simulink model "imcpendel3"  (R2021b)
settings: Solver=ode15s  StartTime=0.0  StopTime=1000  RelTol=1e-3
values from neighbouring files (symbols this model uses):
  A = double(A)    [Eindampfanlage.m]
  B = double(B)    [Eindampfanlage.m]
  C = double(C)    [Eindampfanlage.m]
  D = zeros(p,m)    [Eindampfanlage.m]
  xR = [1; 15; 70]    [Eindampfanlage.m]
settings Model: Creator=mluser  LastModifiedBy=1star
settings DebuggingCC: UnconnectedInputMsg=none  UnconnectedOutputMsg=none  UnconnectedLineMsg=none
settings ModelReferenceCC: EnableRefExpFcnMdlSchedulingChecks=off
settings RTWCC: DLArmComputeVersion=20.02.1

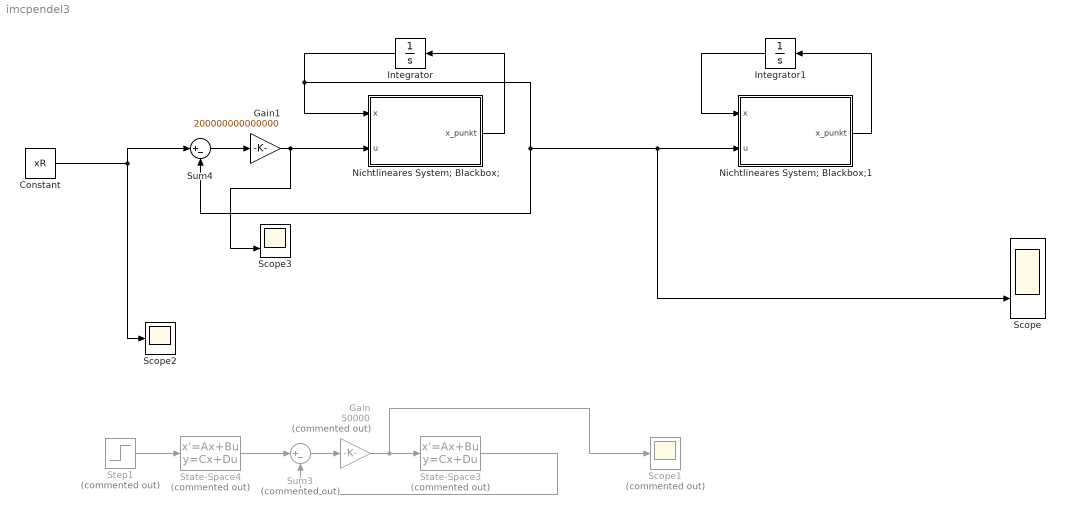
== system imcpendel3 ==
  Constant : Constant  Value=xR
  Gain : Gain  Commented=on  Gain=50000
  Gain1 : Gain  Gain=200000000000000
  Integrator : Integrator  InitialCondition=xR
  Integrator1 : Integrator  InitialCondition=xR
  Nichtlineares System; Blackbox; : MATLAB Function
  Nichtlineares System; Blackbox;1 : MATLAB Function
  Scope : Scope  NumInputPorts=2
  Scope1 : Scope  Commented=on
  Scope2 : Scope
  Scope3 : Scope  NumInputPorts=2
  State-Space3 : StateSpace  Commented=on  A=A  B=B  C=C  D=D  InitialCondition=0
  State-Space4 : StateSpace  Commented=on  A=A  B=B  C=C  D=D  InitialCondition=0
  Step1 : Step  Commented=on  SampleTime=0
  Sum3 : Sum  Commented=on  Inputs=|+-
  Sum4 : Sum  Inputs=|+-
  wires:
  State-Space3/1 -> Sum3/2
  Step1/1 -> State-Space4/1
  State-Space4/1 -> Sum3/1
  Gain/1 -> Scope1/1, State-Space3/1
  Sum3/1 -> Gain/1
  Nichtlineares System; Blackbox;/1(x_punkt) -> Integrator/1
  Constant/1 -> Scope2/1, Sum4/1
  Sum4/1 -> Gain1/1
  Gain1/1 -> Scope3/2, Nichtlineares System; Blackbox;/2(u)
  Integrator/1 -> Scope/2, Nichtlineares System; Blackbox;1/2(u), Sum4/2, Nichtlineares System; Blackbox;/1(x)
  Nichtlineares System; Blackbox;1/1(x_punkt) -> Integrator1/1
  Integrator1/1 -> Nichtlineares System; Blackbox;1/1(x)

== matlab function imcpendel3/Nichtlineares System; Blackbox; ==
  data: x input; x_punkt output; u input
function x_punkt = fcn(x, u)
a1 = 0.00751;
a2 = 0.00418;
a3 = 0.05;
a4 = 0.03755;
a5 = 0.02091;
a6 = 0.00315;

b1 = 0.00192;
b2 = 0.05;
b3 = 0.00959;
b4 = 0.1866;
b5 = 0.14;

k1 = 0.01061;
k2 = 2.5;
k3 = 6.84;
k4 = 2.5531;

x1_punkt = a1*x(3)+a2*x(2)-b1*u(1)-b2*u(2)-k1;
x2_punkt = -a3*x(2)*u(2)+k2;
x3_punkt = -a4*x(3)-a5*x(2)+b3*u(1)-(a6*x(3)+b4)*u(3)/(b5*u(3)+k3)+k4;

x_punkt = [x1_punkt;x2_punkt;x3_punkt];

== matlab function imcpendel3/Nichtlineares System; Blackbox;1 ==
  data: x input; x_punkt output; u input
function x_punkt = fcn(x, u)
a1 = 0.00751;
a2 = 0.00418;
a3 = 0.05;
a4 = 0.03755;
a5 = 0.02091;
a6 = 0.00315;

b1 = 0.00192;
b2 = 0.05;
b3 = 0.00959;
b4 = 0.1866;
b5 = 0.14;

k1 = 0.01061;
k2 = 2.5;
k3 = 6.84;
k4 = 2.5531;

x1_punkt = a1*x(3)+a2*x(2)-b1*u(1)-b2*u(2)-k1;
x2_punkt = -a3*x(2)*u(2)+k2;
x3_punkt = -a4*x(3)-a5*x(2)+b3*u(1)-(a6*x(3)+b4)*u(3)/(b5*u(3)+k3)+k4;

x_punkt = [x1_punkt;x2_punkt;x3_punkt]
